simulink model "rtwdemo_autosar_testharness"  (Simulink 7.6)
settings: Solver=FixedStepDiscrete  StartTime=0.0  StopTime=10.0  FixedStep=0.001  RelTol=1e-3
undefined symbols (not defined in the file or in its folder): sigbuilder_block
settings Model: Creator=The MathWorks Inc.
settings OptimizationCC: InitFltsAndDblsToZero=on  LifeSpan=1
settings DebuggingCC: StrictBusMsg=Warning
settings HardwareCC: ProdIntDivRoundTo=Zero  ProdEndianess=LittleEndian  ProdHWDeviceType=Generic->32-bit Embedded Processor

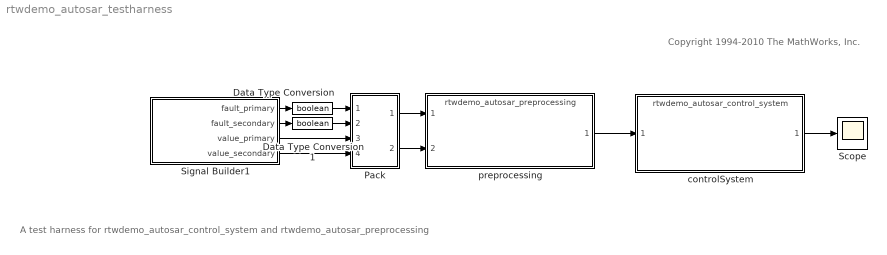
== system rtwdemo_autosar_testharness ==
  note: Copyright 1994-2010 The MathWorks, Inc.
  note: A test harness for rtwdemo_autosar_control_system and rtwdemo_autosar_preprocessing
  Data Type Conversion : DataTypeConversion  OutDataTypeStr=boolean
  Data Type Conversion1 : DataTypeConversion  OutDataTypeStr=boolean
  Pack : Subsystem
  Scope : Scope
      settings: MaxDataPoints=10000
  Signal Builder1 : Subsystem  Tag=STV Subsys  LoadFcn=sigbuilder_block('load');  StartFcn=sigbuilder_block('start');  StopFcn=sigbuilder_block('stop');  ClipboardFcn=sigbuilder_block('clipboard');  mask(Sigbuilder block){}
      mask help: Sigbuilder GUI
      mask init:
      | if ~strcmp(get_param(bdroot(gcbh),'SimulationStatus'),'stopped') tuvar = sigbuilder_block('maskInit'); end
      settings: CopyFcn=sigbuilder_block('copy');  DeleteFcn=sigbuilder_block('delete');  ModelCloseFcn=sigbuilder_block('modelClose');  PreSaveFcn=sigbuilder_block('preSave');  NameChangeFcn=sigbuilder_block('namechange');  OpenFcn=sigbuilder_block('open',[437.6 199.2 550.4 400 ]);  CloseFcn=sigbuilder_block('close');
      mask Display: plot(0,0,100,100,[10,10,40,40,10],[80,20,20,80,80],[40,10],[50,50], [40,27,10],[65,72,56],[40,25,25,10],[28,28,43,43]);
  controlSystem : ModelReference  ModelNameDialog=rtwdemo_autosar_control_system  SimulationMode=Normal  ModelReferenceVersion=1.13  CopyOfModelName=rtwdemo_autosar_control_system
  preprocessing : ModelReference  ModelNameDialog=rtwdemo_autosar_preprocessing  SimulationMode=Normal  ModelReferenceVersion=1.17  CopyOfModelName=rtwdemo_autosar_preprocessing
  wires:
  preprocessing/1 -> controlSystem/1
  controlSystem/1 -> Scope/1
  Signal Builder1/1(fault_primary) -> Data Type Conversion/1
  Signal Builder1/2(fault_secondary) -> Data Type Conversion1/1
  Signal Builder1/3(value_primary) -> Pack/3(value_primary)
  Signal Builder1/4(value_secondary) -> Pack/4(value_secondary)
  Pack/1(faults) -> preprocessing/1
  Pack/2(values) -> preprocessing/2
  Data Type Conversion/1 -> Pack/1(fault_primary)
  Data Type Conversion1/1 -> Pack/2(fault_secondary)

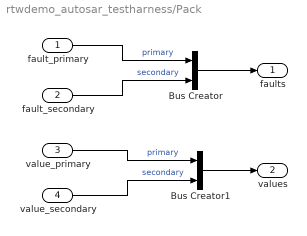
== system rtwdemo_autosar_testharness/Pack ==
  fault_primary : Inport
  fault_secondary : Inport  Port=2
  value_primary : Inport  Port=3
  value_secondary : Inport  Port=4
  Bus Creator : BusCreator  Inputs=2
  Bus Creator1 : BusCreator  Inputs=2
  faults : Outport
  values : Outport  Port=2
  wires:
  fault_primary/1 -> Bus Creator/1  "primary"
  fault_secondary/1 -> Bus Creator/2  "secondary"
  Bus Creator/1 -> faults/1
  value_primary/1 -> Bus Creator1/1  "primary"
  value_secondary/1 -> Bus Creator1/2  "secondary"
  Bus Creator1/1 -> values/1

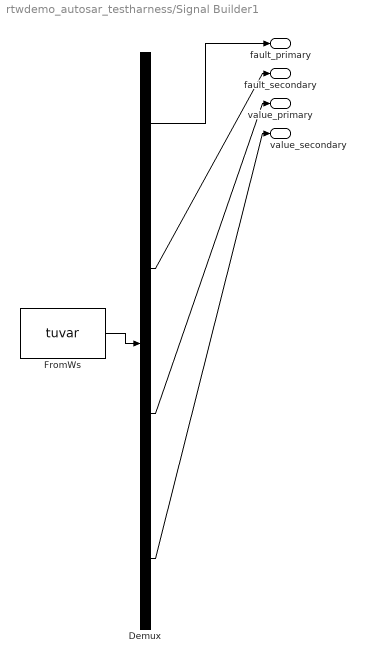
== system rtwdemo_autosar_testharness/Signal Builder1 ==
  Demux : Demux  Tag=STV Demux
  FromWs : FromWorkspace  Tag=STV FromWs  VariableName=tuvar  SampleTime=0.001  SigBuilderData=DataTag0  VnvData=DataTag1
      SigBuilderData=|
      | common.afterFinalStr = 'Extrapolate'
      | common.sampleTime = '0.001'
      | dataSet.timeRange = [0 10]
      | dataSet.name = 'Group 1'
      | sbobj.Name = 'Signal Builder'
      | sbobj.Groups.Name = 'Group 1'
      | sbobj.Groups.Signals(1).Name = 'fault_primary'
      | sbobj.Groups.Signals(1).XData = [0 3 3 5 5 10]
      | sbobj.Groups.Signals(1).YData = [0 0 1 1 0 0]
      | sbobj.Groups.Signals(2).Name = 'fault_secondary'
      | sbobj.Groups.Signals(2).XData = [0 4 4 6 6 10]
      | sbobj.Groups.Signals(2).YData = [0 0 1 1 0 0]
      | sbobj.Groups.Signals(3).Name = 'value_primary'
      | sbobj.Groups.Signals(3).XData = [0 1 1 2 2 3 3 4 4 5 5 6 6 7 7 8 8 9 9 10]
      | sbobj.Groups.Signals(3).YData = [0 2 0 2 0 2 0 2 0 2 0 2 0 2 0 2 0 2 0 2]
      | sbobj.Groups.Signals(4).Name = 'value_secondary'
      | sbobj.Groups.Signals(4).XData = [0 1 1 2 2 3 3 4 4 5 5 6 6 7 7 8 8 9 9 10]
      | sbobj.Groups.Signals(4).YData = [-0.1 2.1 -0.1 2.1 -0.1 2.1 -0.1 2.1 -0.1 2.1 -0.1 2.1 -0.1 2.1 -0.1 2.1 -0.1 2.1 -0.1 2.1]
  fault_primary : Outport  Tag=STV Outport
  fault_secondary : Outport  Tag=STV Outport  Port=2
  value_primary : Outport  Tag=STV Outport  Port=3
  value_secondary : Outport  Tag=STV Outport  Port=4
  wires:
  Demux/1 -> fault_primary/1
  FromWs/1 -> Demux/1
  Demux/2 -> fault_secondary/1
  Demux/3 -> value_primary/1
  Demux/4 -> value_secondary/1
